simulink model "Adaptive_MPC_design"  (R2024b)
settings: Solver=VariableStepAuto  StartTime=0.0  StopTime=300  RelTol=1e-3
values from neighbouring files (symbols this model uses):
  fault_injection = uint8(0)    [Plant_MPC_design.m]    (also in RUNME_CAS781_Project.m)
  VB_table = [      4.4704   1.14   2.29   4.58 ... (first row only)    [Plant_MPC_design.m]
  waypoints_AVa = waypoints_AVa_straight{idx}    [Plant_MPC_design.m]    (also in RUNME_CAS781_Project.m = waypoints_AVa_curved{idx})
  waypoints_AVb = waypoints_AVb_straight{idx}    [Plant_MPC_design.m]    (also in RUNME_CAS781_Project.m = waypoints_AVb_curved{idx})
  y0_AVa = 3    [Plant_MPC_design.m]    (also in RUNME_CAS781_Project.m = 4)
undefined symbols (not defined in the file or in its folder): DiscIntNeverNeededParam
libraries: mpclib x2, Adaptive_Library x2
settings Model: Creator=masra  LastModifiedBy=masra
settings DebuggingCC: UnderSpecifiedDimensionMsg=warning

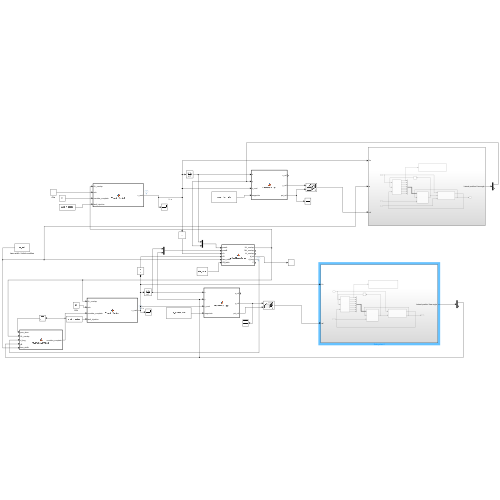
[thumbnail: Simulink's stored preview of the top-level diagram]
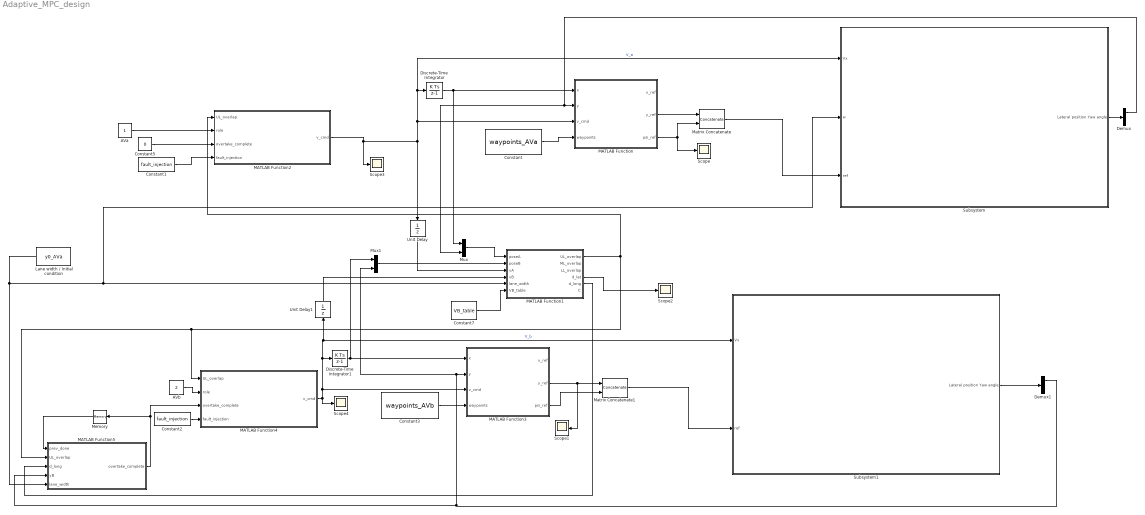
== system Adaptive_MPC_design ==
  AVa : Constant
  AVb : Constant  Value=2
  Constant : Constant  Value=waypoints_AVa
  Constant1 : Constant  Value=fault_injection
  Constant2 : Constant  Value=fault_injection
  Constant3 : Constant  Value=waypoints_AVb
  Constant5 : Constant  Value=0
  Constant7 : Constant  Value=VB_table
  Demux : Demux  Outputs=2
  Demux1 : Demux  Outputs=2
  Discrete-Time Integrator : DiscreteIntegrator  gainval=Ts  SampleTime=-1  ICPrevOutput=DiscIntNeverNeededParam  ICPrevScaledInput=DiscIntNeverNeededParam
  Discrete-Time Integrator1 : DiscreteIntegrator  gainval=Ts  SampleTime=-1  ICPrevOutput=DiscIntNeverNeededParam  ICPrevScaledInput=DiscIntNeverNeededParam
  Lane width / Initial condition : Constant  Value=y0_AVa
  MATLAB Function : MATLAB Function  TreatAsAtomicUnit=on
  MATLAB Function1 : MATLAB Function  TreatAsAtomicUnit=on
  MATLAB Function2 : MATLAB Function  TreatAsAtomicUnit=on
  MATLAB Function3 : MATLAB Function  TreatAsAtomicUnit=on
  MATLAB Function4 : MATLAB Function  TreatAsAtomicUnit=on
  MATLAB Function5 : MATLAB Function  TreatAsAtomicUnit=on
  Matrix Concatenate : Concatenate  Mode=Multidimensional array  ConcatenateDimension=2
  Matrix Concatenate1 : Concatenate  Mode=Multidimensional array  ConcatenateDimension=2
  Memory : Memory
  Mux : Mux  Inputs=2
  Mux1 : Mux  Inputs=2
  Scope{,1..4} (5 alike) : Scope
  Subsystem : Subsystem
  Subsystem1 : Subsystem
  Unit Delay : UnitDelay  SampleTime=-1  HasFrameUpgradeWarning=on
  Unit Delay1 : UnitDelay  SampleTime=-1  HasFrameUpgradeWarning=on
  wires:
  MATLAB Function/2(y_ref) -> Matrix Concatenate/1
  MATLAB Function/3(psi_ref) -> Scope/1, Matrix Concatenate/2
  AVa/1 -> MATLAB Function2/2(role)
  Discrete-Time Integrator/1 -> Mux/1, MATLAB Function/1(x)
  Demux/1 -> Mux/2, MATLAB Function/2(y)
  Matrix Concatenate/1 -> Subsystem/3(ref)
  Subsystem/1(Lateral position Yaw angle) -> Demux/1
  Mux/1 -> MATLAB Function1/1(poseA)
  Constant7/1 -> MATLAB Function1/6(VB_table)
  AVb/1 -> MATLAB Function4/2(role)
  MATLAB Function1/1(UL_overlap) -> MATLAB Function4/1(UL_overlap), MATLAB Function5/2(UL_overlap), MATLAB Function2/1(UL_overlap)
  Discrete-Time Integrator1/1 -> Mux1/1, MATLAB Function3/1(x)
  Subsystem1/1(Lateral position Yaw angle) -> Demux1/1
  Matrix Concatenate1/1 -> Subsystem1/2(ref)
  MATLAB Function3/3(psi_ref) -> Matrix Concatenate1/2
  MATLAB Function3/2(y_ref) -> Scope1/1, Matrix Concatenate1/1
  Mux1/1 -> MATLAB Function1/2(poseB)
  Unit Delay/1 -> MATLAB Function1/3(vA)
  Unit Delay1/1 -> MATLAB Function1/4(vB)
  Constant5/1 -> MATLAB Function2/3(overtake_complete)
  MATLAB Function2/1(v_cmd) -> Subsystem/1(Vx), Discrete-Time Integrator/1, MATLAB Function/3(v_cmd), Unit Delay/1, Scope3/1  "V_a"
  MATLAB Function4/1(v_cmd) -> Scope4/1, Unit Delay1/1, Subsystem1/1(Vx), Discrete-Time Integrator1/1, MATLAB Function3/3(v_cmd)  "V_b"
  MATLAB Function5/1(overtake_complete) -> MATLAB Function4/3(overtake_complete), Memory/1
  Demux1/1 -> Mux1/2, MATLAB Function3/2(y), MATLAB Function5/4(yB)
  MATLAB Function1/5(d_long) -> MATLAB Function5/3(d_long)
  Memory/1 -> MATLAB Function5/1(prev_done)
  MATLAB Function1/4(d_lat) -> Scope2/1
  Lane width / Initial condition/1 -> MATLAB Function5/5(lane_width), Subsystem/2(w), MATLAB Function1/5(lane_width)
  Constant1/1 -> MATLAB Function2/4(fault_injection)
  Constant2/1 -> MATLAB Function4/4(fault_injection)
  Constant/1 -> MATLAB Function/4(waypoints)
  Constant3/1 -> MATLAB Function3/4(waypoints)

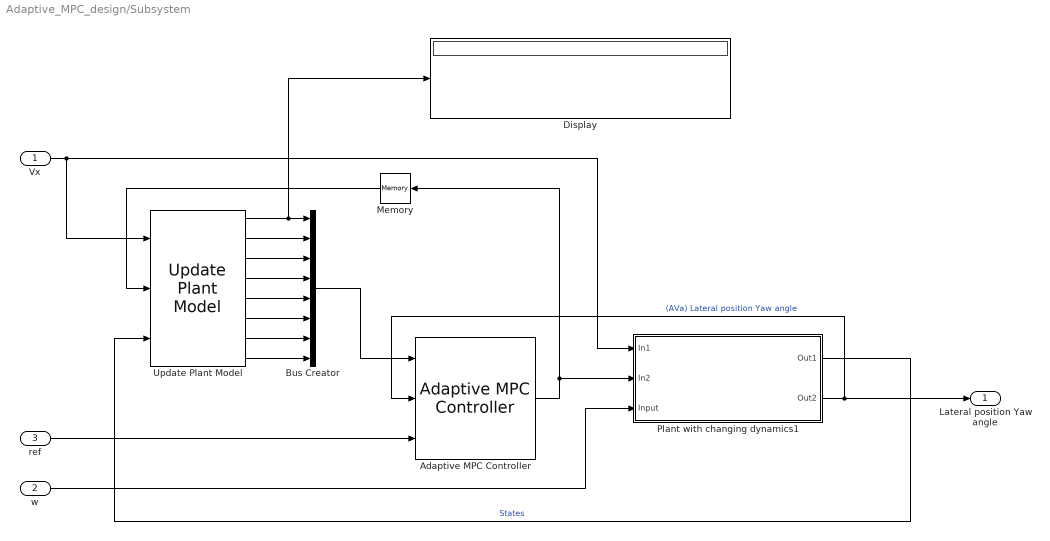
== system Adaptive_MPC_design/Subsystem ==
  Vx : Inport
  w : Inport  Port=2
  ref : Inport  Port=3
  Adaptive MPC Controller : mpclib/Adaptive MPC Controller  SCDEnableBlockLinearizationSpecification=on  mpcobj=mpcobj  x0=x0  enable_value=0  updateMPCinCallerWorkspace=on  md_inport=off  mv_inport=off  uref_inport=off  return_cost=off  return_mvseq=off  return_qpstatus=off  return_xseq=off  return_state=off  return_ovseq=off  state_inport=off  isltv_plant=off  umin_inport=off  umax_inport=off  ymin_inport=off  ymax_inport=off  cc_inport=off  ywt_inport=off  uwt_inport=off  duwt_inport=off  rhoeps_inport=off  pm_inport=off  MaximumP=10  HorizonChoice=FixedHorizon  BlockDataType=double  SampleTimeInherited=off  switch_inport=off
  Bus Creator : BusCreator  Inputs=8
  Display : Display
  Memory : Memory
  Plant with changing dynamics1 : Subsystem  AncestorBlock=Adaptive_Library/Plant with changing dynamics1
      mask Display: image('car.jpg');
  Update Plant Model : Adaptive_Library/Update Plant Model  SystemSampleTime=-1  VariantActivationTime=update diagram  AllowFlexibleInterface=on  Latency=0  AutoFrameSizeCalculation=off
  Lateral position Yaw angle : Outport
  wires:
  Update Plant Model/1 -> Display/1, Bus Creator/1
  Update Plant Model/8 -> Bus Creator/8
  Plant with changing dynamics1/2(Out2) -> Lateral position Yaw angle/1, Adaptive MPC Controller/2  "(AVa) Lateral position Yaw angle"
  Update Plant Model/5 -> Bus Creator/5
  Bus Creator/1 -> Adaptive MPC Controller/1
  Plant with changing dynamics1/1(Out1) -> Update Plant Model/3  "States"
  Memory/1 -> Update Plant Model/2
  Vx/1 -> Update Plant Model/1, Plant with changing dynamics1/1(In1)
  Update Plant Model/3 -> Bus Creator/3
  Update Plant Model/7 -> Bus Creator/7
  Adaptive MPC Controller/1 -> Plant with changing dynamics1/2(In2), Memory/1
  Update Plant Model/6 -> Bus Creator/6
  Update Plant Model/4 -> Bus Creator/4
  Update Plant Model/2 -> Bus Creator/2
  ref/1 -> Adaptive MPC Controller/3
  w/1 -> Plant with changing dynamics1/3(Input)

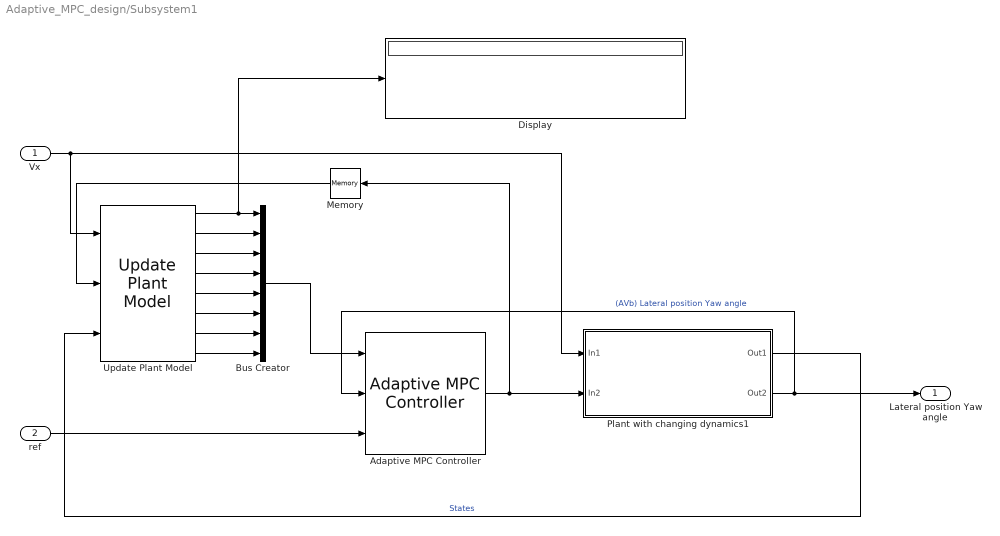
== system Adaptive_MPC_design/Subsystem1 ==
  Vx : Inport
  ref : Inport  Port=2
  Adaptive MPC Controller : mpclib/Adaptive MPC Controller  SCDEnableBlockLinearizationSpecification=on  mpcobj=mpcobj  enable_value=0  updateMPCinCallerWorkspace=on  md_inport=off  mv_inport=off  uref_inport=off  return_cost=off  return_mvseq=off  return_qpstatus=off  return_xseq=off  return_state=off  return_ovseq=off  state_inport=off  isltv_plant=off  umin_inport=off  umax_inport=off  ymin_inport=off  ymax_inport=off  cc_inport=off  ywt_inport=off  uwt_inport=off  duwt_inport=off  rhoeps_inport=off  pm_inport=off  MaximumP=10  HorizonChoice=FixedHorizon  BlockDataType=double  SampleTimeInherited=off  switch_inport=off
  Bus Creator : BusCreator  Inputs=8
  Display : Display
  Memory : Memory
  Plant with changing dynamics1 : Subsystem  AncestorBlock=Adaptive_Library/Plant with changing dynamics1
      mask Display: image('car.jpg');
  Update Plant Model : Adaptive_Library/Update Plant Model  SystemSampleTime=-1  VariantActivationTime=update diagram  AllowFlexibleInterface=on  Latency=0  AutoFrameSizeCalculation=off
  Lateral position Yaw angle : Outport
  wires:
  Update Plant Model/1 -> Display/1, Bus Creator/1
  Update Plant Model/8 -> Bus Creator/8
  Plant with changing dynamics1/2(Out2) -> Lateral position Yaw angle/1, Adaptive MPC Controller/2  "(AVb) Lateral position Yaw angle"
  Update Plant Model/5 -> Bus Creator/5
  Bus Creator/1 -> Adaptive MPC Controller/1
  Plant with changing dynamics1/1(Out1) -> Update Plant Model/3  "States"
  Memory/1 -> Update Plant Model/2
  Vx/1 -> Plant with changing dynamics1/1(In1), Update Plant Model/1
  Update Plant Model/3 -> Bus Creator/3
  Update Plant Model/7 -> Bus Creator/7
  Adaptive MPC Controller/1 -> Plant with changing dynamics1/2(In2), Memory/1
  Update Plant Model/6 -> Bus Creator/6
  Update Plant Model/4 -> Bus Creator/4
  Update Plant Model/2 -> Bus Creator/2
  ref/1 -> Adaptive MPC Controller/3

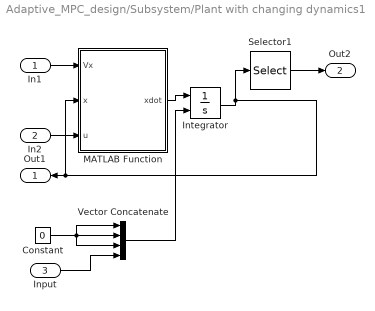
== system Adaptive_MPC_design/Subsystem/Plant with changing dynamics1 ==
  In1 : Inport
  In2 : Inport  Port=2
  Input : Inport  Port=3
  Constant : Constant  Value=0
  Integrator : Integrator  InitialConditionSource=external  InitialCondition=[0; 0; 0; 3]
  MATLAB Function : MATLAB Function  TreatAsAtomicUnit=on
  Selector1 : Selector  InputPortWidth=4  IndexOptions=Index vector (dialog)  Indices=[4 2]  OutputSizes=1
  Vector Concatenate : Concatenate  NumInputs=4
  Out1 : Outport  VectorParamsAs1DForOutWhenUnconnected=off
  Out2 : Outport  Port=2  VectorParamsAs1DForOutWhenUnconnected=off
  wires:
  Selector1/1 -> Out2/1
  MATLAB Function/1(xdot) -> Integrator/1
  Integrator/1 -> Out1/1, MATLAB Function/2(x), Selector1/1
  In1/1 -> MATLAB Function/1(Vx)
  In2/1 -> MATLAB Function/3(u)
  Input/1 -> Vector Concatenate/4
  Constant/1 -> Vector Concatenate/1, Vector Concatenate/3, Vector Concatenate/2
  Vector Concatenate/1 -> Integrator/2

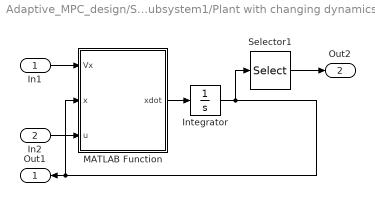
== system Adaptive_MPC_design/Subsystem1/Plant with changing dynamics1 ==
  In1 : Inport
  In2 : Inport  Port=2
  Integrator : Integrator  InitialCondition=[0; 0; 0; 0]
  MATLAB Function : MATLAB Function  TreatAsAtomicUnit=on
  Selector1 : Selector  InputPortWidth=4  IndexOptions=Index vector (dialog)  Indices=[4 2]  OutputSizes=1
  Out1 : Outport  VectorParamsAs1DForOutWhenUnconnected=off
  Out2 : Outport  Port=2  VectorParamsAs1DForOutWhenUnconnected=off
  wires:
  Selector1/1 -> Out2/1
  MATLAB Function/1(xdot) -> Integrator/1
  Integrator/1 -> Out1/1, MATLAB Function/2(x), Selector1/1
  In1/1 -> MATLAB Function/1(Vx)
  In2/1 -> MATLAB Function/3(u)

== matlab function Adaptive_MPC_design/Subsystem1/Plant with changing dynamics1/MATLAB Function ==
  data: Vx input; x input size=[4,1]; u input; xdot output size=[4,1]
function xdot = fcn(Vx,x,u)

% Model parameters
m = 1575;
Iz = 2875;
lf = 1.2;
lr = 1.6;
Cf = 19000;
Cr = 33000;

% Continuous-time model
A = [-(2*Cf+2*Cr)/m/Vx, 0, -Vx-(2*Cf*lf-2*Cr*lr)/m/Vx, 0;
     0, 0, 1, 0;
     -(2*Cf*lf-2*Cr*lr)/Iz/Vx, 0, -(2*Cf*lf^2+2*Cr*lr^2)/Iz/Vx, 0;
     1, Vx, 0, 0];
B = [2*Cf/m 0 2*Cf*lf/Iz 0]';   
C = [0 0 0 1; 0 1 0 0];
D = zeros(2,1);
xdot = A*x + B*u;
%y = C*x + D*u;

== matlab function Adaptive_MPC_design/MATLAB Function1 ==
  settings: updateMethod=DISCRETE
  data: poseA input size=[2]; UL_overlap output; poseB input size=[2]; vA input; vB input; lane_width input; VB_table input size=[4 4]; ML_overlap output; LL_overlap output; d_lat output; d_long output; C output
function [UL_overlap, ML_overlap, LL_overlap, d_lat, d_long, C] = ...
    VirtualBoundaries(poseA, poseB, vA, vB, lane_width, VB_table)
%#codegen
% poseA, poseB : [x; y] positions of AVa and AVb in global coordinates
% vA, vB       : scalar speeds (m/s)
% lane_width   : lane width (m) – not directly used below
% VB_table     : [v  LL  ML  UL] lookup table (rows: speeds)
%
% Outputs
%   UL_overlap, ML_overlap, LL_overlap : VB overlap flags (for logic)
%   d_lat, d_long                      : lateral / longitudinal separations
%   C                                  : relative collision metric (eq. 3)

    % ---- lateral side VBs ----
    % You can make these depend on lane_width if you want.
    S_a = lane_width/2;     % [m] side VB for AVa
    S_b = lane_width/2;     % [m] side VB for AVb

    % ---- signed separations (eq. 1 & 2) ----
    y_s = poseB(2) - poseA(2);   % lateral separation (B relative to A)
    x_s = poseB(1) - poseA(1);   % longitudinal separation

    d_lat  = abs(y_s);
    d_long = x_s;                % keep sign for logging
    d_long_abs = abs(x_s);
    d_lat_abs  = abs(y_s);

    % ---- lookup longitudinal VB distances from table ----
    speeds = VB_table(:,1);      % first column: speed in m/s

    [~, idxA] = min(abs(speeds - vA));
    [~, idxB] = min(abs(speeds - vB));

    LL_A = VB_table(idxA,2);
    ML_A = VB_table(idxA,3);
    UL_A = VB_table(idxA,4);

    LL_B = VB_table(idxB,2);
    ML_B = VB_table(idxB,3);
    UL_B = VB_table(idxB,4);

    U_long = UL_A + UL_B;        % U_af + U_br
    M_long = ML_A + ML_B;
    L_long = LL_A + LL_B;
    S_side = S_a + S_b;          % S_bl + S_ar

    % ============================================================
    %   1) RAW GEOMETRIC OVERLAP FLAGS (no hysteresis)
    % ============================================================
    UL_raw = (d_long_abs <= U_long);
    ML_raw = (d_long_abs <= M_long);
    LL_raw = (d_long_abs <= L_long);

    % if lateral separation exceeds side VBs, no overlap at all
    if d_lat_abs > S_side
        UL_raw = false;
        ML_raw = false;
        LL_raw = false;
    end

    % ============================================================
    %   2) RELATIVE COLLISION METRIC C (equation 3)
    % ============================================================
    % By construction, C_raw = 0 outside the VB regions.
    C_raw = 0;

    if UL_raw || ML_raw || LL_raw
        % longitudinal term [1 - x_s/(U_af+U_br)]^+
        if U_long > 0
            gamma_long = 1 - d_long_abs / U_long;
        else
            gamma_long = 0;
        end
        gamma_long = max(0, min(1, gamma_long));

        % lateral term [1 - y_s/(S_bl+S_ar)]^+
        if S_side > 0
            gamma_lat = 1 - d_lat_abs / S_side;
        else
            gamma_lat = 0;
        end
        gamma_lat = max(0, min(1, gamma_lat));

        C_raw = gamma_long * gamma_lat;
    end

    % Clamp to [0,1] just in case of numerical noise
    C_raw = max(0, min(1, C_raw));

    epsC_raw = 6.3e-3;
    if C_raw < epsC_raw
        C_raw = 0;
    end


    % This is the value you plot
    C = C_raw;

    % ============================================================
    %   3) HYSTERESIS ON C TO DEFINE UL_overlap
    % ============================================================
    % We use C as a risk indicator and introduce hysteresis to avoid
    % chattering around C ≈ 0:
    %   - when C rises above C_on  -> UL_overlap becomes true
    %   - when C falls below C_off -> UL_overlap becomes false
    % with C_off < C_on.
    persistent UL_flag
    if isempty(UL_flag)
        UL_flag = false;
    end

    C_on  = 1e-3;   % enter overlap region
    C_off = 5e-4;   % leave overlap region (must be < C_on)

    if UL_flag
        % currently in overlap state
        if C_raw < C_off
            UL_flag = false;
        end
    else
        % currently outside overlap, only enter if clearly non-zero
        if C_raw > C_on
            UL_flag = true;
        end
    end

    UL_overlap = UL_flag;

    % For now ML/LL can simply mirror the raw flags
    ML_overlap = ML_raw;
    LL_overlap = LL_raw;
end

== matlab function Adaptive_MPC_design/MATLAB Function ==
  data: x_ref output; x input size=1; y input size=1; y_ref output size=20, 1; psi_ref output size=20, 1; v_cmd input; waypoints input
function [x_ref, y_ref, psi_ref] = ReferenceLogic(x, y, v_cmd, waypoints)
%#codegen
% Generate a H-step reference trajectory from a global waypoint path.
%
% Inputs:
%   x, y      : current vehicle position [m]
%   v_cmd     : commanded longitudinal speed [m/s]
%   waypoints : N x 2 matrix [wx wy] representing the global path [m]
%
% Outputs:
%   x_ref, y_ref, psi_ref : H x 1 vectors of reference pose for MPC

    % Prediction horizon and sampling time (must match the MPC setup)
    H  = 20;     % prediction horizon
    Ts = 0.1;    % sampling time [s]

    % Preallocate outputs with fixed size for code generation
    x_ref  = zeros(H,1);
    y_ref  = zeros(H,1);
    psi_ref = zeros(H,1);

    % Guard: if we don't have a valid path, hold the current pose
    N = size(waypoints,1);
    if N < 2
        for k = 1:H
            x_ref(k)  = x;
            y_ref(k)  = y;
            psi_ref(k) = 0.0;
        end
        return;
    end

    % --- build cumulative arc-length of path ---
    wx = waypoints(:,1);
    wy = waypoints(:,2);

    s = zeros(N,1);
    for i = 2:N
        dx = wx(i) - wx(i-1);
        dy = wy(i) - wy(i-1);
        s(i) = s(i-1) + sqrt(dx*dx + dy*dy);
    end

    % --- find closest point on path to (x,y) ---
    % (nearest Euclidean distance)
    min_dist2 = inf;
    idx_closest = 1;
    for i = 1:N
        dx = wx(i) - x;
        dy = wy(i) - y;
        dist2 = dx*dx + dy*dy;
        if dist2 < min_dist2
            min_dist2 = dist2;
            idx_closest = i;
        end
    end

    % Arc-length at projection of (x,y) on the path
    if idx_closest < N
        p1x = wx(idx_closest);
        p1y = wy(idx_closest);
        p2x = wx(idx_closest+1);
        p2y = wy(idx_closest+1);

        vx_seg = p2x - p1x;
        vy_seg = p2y - p1y;
        seg_norm2 = vx_seg*vx_seg + vy_seg*vy_seg;

        if seg_norm2 < 1e-8
            alpha = 0.0;
        else
            px = x - p1x;
            py = y - p1y;
            alpha = (px*vx_seg + py*vy_seg) / seg_norm2;
            if alpha < 0.0
                alpha = 0.0;
            elseif alpha > 1.0
                alpha = 1.0;
            end
        end

        seg_len = sqrt(vx_seg*vx_seg + vy_seg*vy_seg);
        s0 = s(idx_closest) + alpha * seg_len;
    else
        s0 = s(end);
    end

    % --- future arc-lengths (assume constant v_cmd over horizon) ---
    s_future = zeros(H,1);
    for k = 1:H
        s_step = s0 + (k-1) * v_cmd * Ts;
        % clamp within path limits
        if s_step < s(1)
            s_step = s(1);
        elseif s_step > s(end)
            s_step = s(end);
        end
        s_future(k) = s_step;
    end

    % --- interpolate positions along the path ---
    xq = interp1(s, wx, s_future, 'linear', 'extrap');
    yq = interp1(s, wy, s_future, 'linear', 'extrap');

    % --- orientation from local tangent ---
    % psi_ref(k) is heading angle at s_future(k)
    for k = 1:H
        sf2 = s_future(k) + 0.01;  % small forward step for tangent
        if sf2 > s(end)
            sf2 = s(end);
        end
        xf2 = interp1(s, wx, sf2, 'linear', 'extrap');
        yf2 = interp1(s, wy, sf2, 'linear', 'extrap');

        dx_t = xf2 - xq(k);
        dy_t = yf2 - yq(k);
        psi_ref(k) = atan2(dy_t, dx_t);
    end

    % assign outputs (ensures fixed-size vectors)
    x_ref = xq;
    y_ref = yq;
end

== matlab function Adaptive_MPC_design/MATLAB Function2 ==
  data: v_cmd output; UL_overlap input; role input; overtake_complete input; fault_injection input size=1
function v_cmd = VelocityControl(UL_overlap, role, overtake_complete, fault_injection)
%#codegen
% VelocityControl implements the deontological velocity rules
% described in the paper for AVa and AVb.
%
% Inputs:
%   UL_overlap       : true if UL virtual boundaries of AVa/AVb overlap
%   role             : 'A' for AVa, 'B' for AVb
%   overtake_complete: true when AVb has safely completed the overtake
%
% Output:
%   v_cmd : commanded longitudinal speed [m/s]

    % Paper parameters (m/s)
    v_A_nom     = 26.82;  % 60 mph, AVa nominal speed in slow lane
    v_A_reduced = 24.59;  % 55 mph, AVa reduced speed if UL not respected
    v_B_nom     = 31.29;  % 70 mph, AVb nominal speed in fast/overtaking lane
    v_B_after   = 26.82;  % 60 mph, AVb speed after completing the overtake

    if role == 1
        if fault_injection == 0
            % AVa: maintain 60 mph unless UL VB is not respected
            if UL_overlap
                % UL not respected -> decelerate to 55 mph
                v_cmd = v_A_reduced;
            else
                % UL respected -> nominal 60 mph
                v_cmd = v_A_nom;
            end
        else
            v_cmd = v_A_nom;
        end

    else
        if fault_injection == 0
            % AVb: keep 70 mph until overtake is complete and ULs are respected,
            % then decelerate to 60 mph in Lane 1.
            if overtake_complete
                v_cmd = v_B_after;
            else
                v_cmd = v_B_nom;
            end
        else
            v_cmd = v_B_nom;
        end
    end
end

== matlab function Adaptive_MPC_design/MATLAB Function3 ==
  data: x_ref output; x input size=1; y input size=1; y_ref output size=20, 1; psi_ref output size=20, 1; v_cmd input; waypoints input
function [x_ref, y_ref, psi_ref] = ReferenceLogic(x, y, v_cmd, waypoints)
%#codegen
% Generate a H-step reference trajectory from a global waypoint path.
%
% Inputs:
%   x, y      : current vehicle position [m]
%   v_cmd     : commanded longitudinal speed [m/s]
%   waypoints : N x 2 matrix [wx wy] representing the global path [m]
%
% Outputs:
%   x_ref, y_ref, psi_ref : H x 1 vectors of reference pose for MPC

    % Prediction horizon and sampling time (must match the MPC setup)
    H  = 20;     % prediction horizon
    Ts = 0.1;    % sampling time [s]

    % Preallocate outputs with fixed size for code generation
    x_ref  = zeros(H,1);
    y_ref  = zeros(H,1);
    psi_ref = zeros(H,1);

    % Guard: if we don't have a valid path, hold the current pose
    N = size(waypoints,1);
    if N < 2
        for k = 1:H
            x_ref(k)  = x;
            y_ref(k)  = y;
            psi_ref(k) = 0.0;
        end
        return;
    end

    % --- build cumulative arc-length of path ---
    wx = waypoints(:,1);
    wy = waypoints(:,2);

    s = zeros(N,1);
    for i = 2:N
        dx = wx(i) - wx(i-1);
        dy = wy(i) - wy(i-1);
        s(i) = s(i-1) + sqrt(dx*dx + dy*dy);
    end

    % --- find closest point on path to (x,y) ---
    % (nearest Euclidean distance)
    min_dist2 = inf;
    idx_closest = 1;
    for i = 1:N
        dx = wx(i) - x;
        dy = wy(i) - y;
        dist2 = dx*dx + dy*dy;
        if dist2 < min_dist2
            min_dist2 = dist2;
            idx_closest = i;
        end
    end

    % Arc-length at projection of (x,y) on the path
    if idx_closest < N
        p1x = wx(idx_closest);
        p1y = wy(idx_closest);
        p2x = wx(idx_closest+1);
        p2y = wy(idx_closest+1);

        vx_seg = p2x - p1x;
        vy_seg = p2y - p1y;
        seg_norm2 = vx_seg*vx_seg + vy_seg*vy_seg;

        if seg_norm2 < 1e-8
            alpha = 0.0;
        else
            px = x - p1x;
            py = y - p1y;
            alpha = (px*vx_seg + py*vy_seg) / seg_norm2;
            if alpha < 0.0
                alpha = 0.0;
            elseif alpha > 1.0
                alpha = 1.0;
            end
        end

        seg_len = sqrt(vx_seg*vx_seg + vy_seg*vy_seg);
        s0 = s(idx_closest) + alpha * seg_len;
    else
        s0 = s(end);
    end

    % --- future arc-lengths (assume constant v_cmd over horizon) ---
    s_future = zeros(H,1);
    for k = 1:H
        s_step = s0 + (k-1) * v_cmd * Ts;
        % clamp within path limits
        if s_step < s(1)
            s_step = s(1);
        elseif s_step > s(end)
            s_step = s(end);
        end
        s_future(k) = s_step;
    end

    % --- interpolate positions along the path ---
    xq = interp1(s, wx, s_future, 'linear', 'extrap');
    yq = interp1(s, wy, s_future, 'linear', 'extrap');

    % --- orientation from local tangent ---
    % psi_ref(k) is heading angle at s_future(k)
    for k = 1:H
        sf2 = s_future(k) + 0.01;  % small forward step for tangent
        if sf2 > s(end)
            sf2 = s(end);
        end
        xf2 = interp1(s, wx, sf2, 'linear', 'extrap');
        yf2 = interp1(s, wy, sf2, 'linear', 'extrap');

        dx_t = xf2 - xq(k);
        dy_t = yf2 - yq(k);
        psi_ref(k) = atan2(dy_t, dx_t);
    end

    % assign outputs (ensures fixed-size vectors)
    x_ref = xq;
    y_ref = yq;
end

== matlab function Adaptive_MPC_design/MATLAB Function4 ==
  data: v_cmd output; UL_overlap input; role input; overtake_complete input; fault_injection input size=1
function v_cmd = VelocityControl(UL_overlap, role, overtake_complete, fault_injection)
%#codegen
% VelocityControl implements the deontological velocity rules
% described in the paper for AVa and AVb.
%
% Inputs:
%   UL_overlap       : true if UL virtual boundaries of AVa/AVb overlap
%   role             : 'A' for AVa, 'B' for AVb
%   overtake_complete: true when AVb has safely completed the overtake
%
% Output:
%   v_cmd : commanded longitudinal speed [m/s]

    % Paper parameters (m/s)
    v_A_nom     = 26.82;  % 60 mph, AVa nominal speed in slow lane
    v_A_reduced = 24.59;  % 55 mph, AVa reduced speed if UL not respected
    v_B_nom     = 31.29;  % 70 mph, AVb nominal speed in fast/overtaking lane
    v_B_after   = 26.82;  % 60 mph, AVb speed after completing the overtake

    if role == 1
        if fault_injection == 0
            % AVa: maintain 60 mph unless UL VB is not respected
            if UL_overlap
                % UL not respected -> decelerate to 55 mph
                v_cmd = v_A_reduced;
            else
                % UL respected -> nominal 60 mph
                v_cmd = v_A_nom;
            end
        else
            v_cmd = v_A_nom;
        end

    else
        if fault_injection == 0
            % AVb: keep 70 mph until overtake is complete and ULs are respected,
            % then decelerate to 60 mph in Lane 1.
            if overtake_complete
                v_cmd = v_B_after;
            else
                v_cmd = v_B_nom;
            end
        else
            v_cmd = v_B_nom;
        end
    end
end

== matlab function Adaptive_MPC_design/MATLAB Function5 ==
  data: prev_done input boolean; UL_overlap input; overtake_complete output; d_long input; yB input; lane_width input
function overtake_complete = OvertakeComplete(prev_done, UL_overlap, d_long, yB, lane_width)
%#codegen
% prev_done    : previous overtake_complete (from Unit Delay)
% UL_overlap   : true if UL VBs overlap
% d_long       : xB - xA
% yB           : lateral position of AVb
% lane_width   : lane width (fast lane centered at y = lane_width)

    % --- condition 1: AVb est en voie rapide (voie du haut) ---
    fast_center = lane_width;          % centre de la voie 2
    lat_tol     = 0.25 * lane_width;   % tolérance : 25% de la largeur de voie
    inFastLane  = abs(yB - fast_center) <= lat_tol;

    % --- condition 2: AVb est bien devant AVa ET plus d'UL overlap ---
    safeMargin   = 10;                 % [m] marge de sécurité
    aheadAndClear = (d_long > safeMargin) && (~UL_overlap);

    % --- latch : une fois vrai, reste vrai ---
    overtake_complete = prev_done || (inFastLane && aheadAndClear);
end

== matlab function Adaptive_MPC_design/Subsystem/Plant with changing dynamics1/MATLAB Function ==
  data: Vx input; x input size=[4,1]; u input; xdot output size=[4,1]
function xdot = fcn(Vx,x,u)

% Model parameters
m = 1575;
Iz = 2875;
lf = 1.2;
lr = 1.6;
Cf = 19000;
Cr = 33000;

% Continuous-time model
A = [-(2*Cf+2*Cr)/m/Vx, 0, -Vx-(2*Cf*lf-2*Cr*lr)/m/Vx, 0;
     0, 0, 1, 0;
     -(2*Cf*lf-2*Cr*lr)/Iz/Vx, 0, -(2*Cf*lf^2+2*Cr*lr^2)/Iz/Vx, 0;
     1, Vx, 0, 0];
B = [2*Cf/m 0 2*Cf*lf/Iz 0]';   
C = [0 0 0 1; 0 1 0 0];
D = zeros(2,1);
xdot = A*x + B*u;
%y = C*x + D*u;
